simulink subsystem "Rectifier_VR_openloop"  (R2024b)
settings: Solver=VariableStepAuto  StartTime=0.0  StopTime=10.0  RelTol=1e-3
settings Model: DataDictionary=RectData.sldd  EnableAccessToBaseWorkspace=off  Creator=sgade  LastModifiedBy=sgade

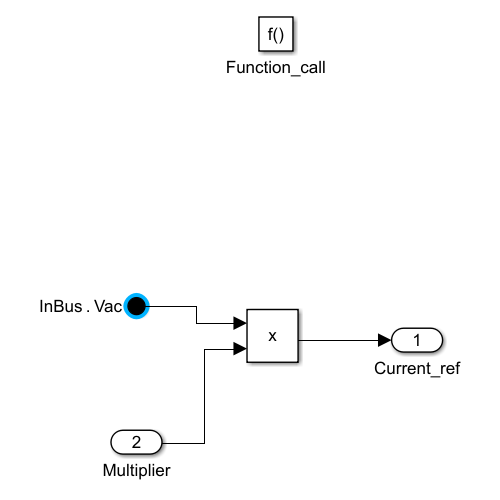
[thumbnail: Simulink's stored preview of the top-level diagram]
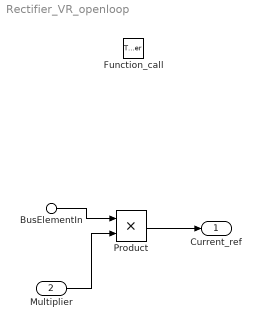
== system Rectifier_VR_openloop ==
  BusElementIn : Inport  PortName=Scaled  Element=Vac
  Multiplier : Inport  Port=2
  Function_call : TriggerPort  TriggerType=function-call  VariantControl=(inherit)  PortDimensions=1
  Product : Product
  Current_ref : Outport
  wires:
  BusElementIn/1 -> Product/1
  Multiplier/1 -> Product/2
  Product/1 -> Current_ref/1
